simulink model "LKS_1"  (R2018a)
settings: Solver=FixedStepAuto  StartTime=0.0  StopTime=10.0  RelTol=1e-3
values from neighbouring files (symbols this model uses):
  a11 = -2*(cf+cr)/m/v    (= -8.91428571429)    [LKS.m]
  a12 = -1-2*(lf*cf-lr*cr)/m/v/v    (= -0.975808)    [LKS.m]
  a21 = -2*(lf*cf-lr*cr)/iz    (= 12.3270440252)    [LKS.m]
  a22 = -2*(lf*lf*cf+lr*lr*cr)/iz/v    (= -9.16473962264)    [LKS.m]
  b11 = 2*cf/m/v    (= 3.42857142857)    [LKS.m]
  b12 = 0    [LKS.m]
  b21 = 2*lf*cf/iz    (= 94.3396226415)    [LKS.m]
  b22 = 1/iz    (= 0.0062893081761)    [LKS.m]
  dv = 0.814    [LKS.m]
  g1 = 2*(cf+cr)/m/v+2*(lf*lf*cf+lr*lr*cr)/iz/v    (= 18.0790253369)    [LKS.m]
  go = 4*l*l*cf*cr/m/iz/v/v-2*(lf*cf-lr*cr)/iz    (= 93.7259356694)    [LKS.m]
  hm1 = 1/iz    (= 0.0062893081761)    [LKS.m]
  hmo = 2*(cf+cr)/m/iz/v    (= 0.056064690027)    [LKS.m]
  L = 6.31    [LKS.m]
  mydt = 0.01    [LKS.m]
  rw = 0.225    [LKS.m]
  v = vkm/3.6    (= 13.8888888889)    [LKS.m]
libraries: simulink x2
settings Model: Creator=aoki-soya  LastModifiedBy=aoki-soya

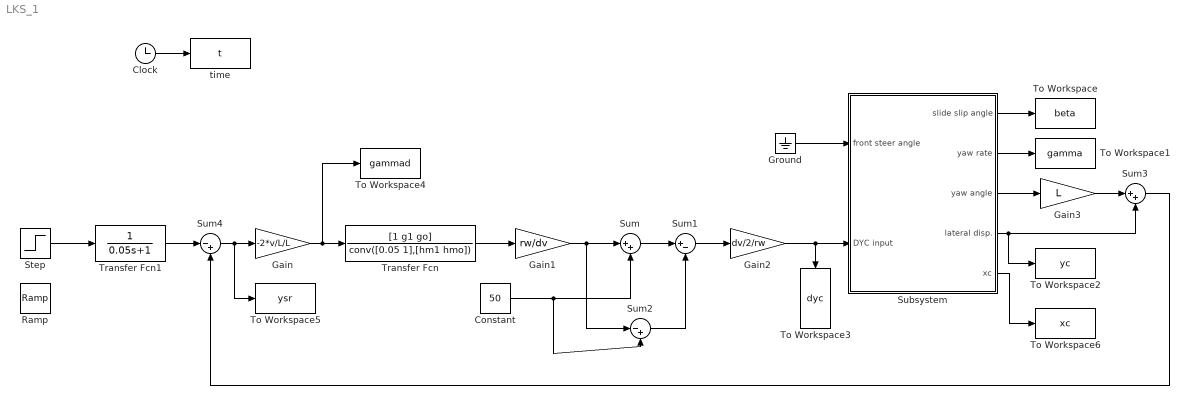
== system LKS_1 ==
  Clock : Clock
      settings: Decimation=1/mydt
  Constant : Constant  Value=50
  Gain : Gain  Gain=-2*v/L/L
  Gain1 : Gain  Gain=rw/dv
  Gain2 : Gain  Gain=dv/2/rw
  Gain3 : Gain  Gain=L
  Ground : Ground
  Ramp : simulink/Sources/Ramp  slope=1  start=1  InitialOutput=0
  Step : Step  SampleTime=mydt
  Subsystem : Subsystem
  Sum : Sum  Inputs=|++
  Sum1 : Sum  Inputs=|+-
  Sum2 : Sum  Inputs=|-+
  Sum3 : Sum  Inputs=|++
  Sum4 : Sum  Inputs=|-+
  To Workspace : ToWorkspace  VariableName=beta  SaveFormat=Timeseries  SampleTime=-1
  To Workspace1 : ToWorkspace  VariableName=gamma  SaveFormat=Timeseries  SampleTime=-1
  To Workspace2 : ToWorkspace  VariableName=yc  SaveFormat=Timeseries  SampleTime=-1
  To Workspace3 : ToWorkspace  VariableName=dyc  SaveFormat=Timeseries  SampleTime=-1
  To Workspace4 : ToWorkspace  VariableName=gammad  SaveFormat=Timeseries  SampleTime=-1
  To Workspace5 : ToWorkspace  VariableName=ysr  SaveFormat=Timeseries  SampleTime=-1
  To Workspace6 : ToWorkspace  VariableName=xc  SaveFormat=Timeseries  SampleTime=-1
  Transfer Fcn : TransferFcn  Numerator=[1 g1 go]  Denominator=conv([0.05 1],[hm1 hmo])
  Transfer Fcn1 : TransferFcn  Denominator=[0.05 1]
  time : ToWorkspace  VariableName=t  SaveFormat=Timeseries  SampleTime=-1
  wires:
  Gain/1 -> To Workspace4/1, Transfer Fcn/1
  Transfer Fcn/1 -> Gain1/1
  Gain1/1 -> Sum2/1, Sum/1
  Sum/1 -> Sum1/1
  Sum2/1 -> Sum1/2
  Constant/1 -> Sum2/2, Sum/2
  Sum1/1 -> Gain2/1
  Gain2/1 -> To Workspace3/1, Subsystem/2(DYC input)
  Ground/1 -> Subsystem/1(front steer angle)
  Clock/1 -> time/1
  Subsystem/3(yaw angle) -> Gain3/1
  Gain3/1 -> Sum3/1
  Sum4/1 -> To Workspace5/1, Gain/1
  Sum3/1 -> Sum4/2
  Subsystem/1(slide slip angle) -> To Workspace/1
  Subsystem/2(yaw rate) -> To Workspace1/1
  Subsystem/4("lateral disp. ") -> To Workspace2/1, Sum3/2
  Subsystem/5("xc ") -> To Workspace6/1
  Transfer Fcn1/1 -> Sum4/1
  Step/1 -> Transfer Fcn1/1

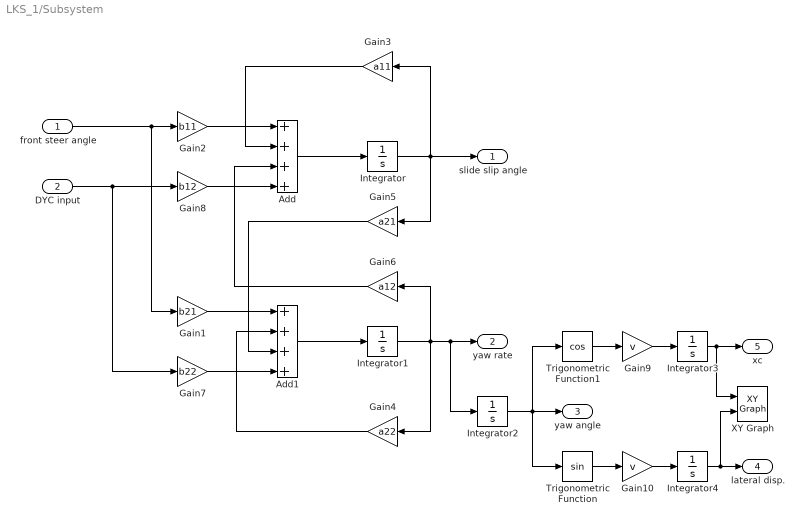
== system LKS_1/Subsystem ==
  front steer angle : Inport
  DYC input : Inport  Port=2
  Add : Sum  Inputs=++++
  Add1 : Sum  Inputs=++++
  Gain1 : Gain  Gain=b21
  Gain10 : Gain  Gain=v
  Gain2 : Gain  Gain=b11
  Gain3 : Gain  Gain=a11
  Gain4 : Gain  Gain=a22
  Gain5 : Gain  Gain=a21
  Gain6 : Gain  Gain=a12
  Gain7 : Gain  Gain=b22
  Gain8 : Gain  Gain=b12
  Gain9 : Gain  Gain=v
  Integrator{,1..4} (5 alike) : Integrator
  Trigonometric Function : Trigonometry
  Trigonometric Function1 : Trigonometry  Operator=cos
  XY Graph : simulink/Sinks/XY Graph  xmin=0  xmax=100  ymin=0  ymax=5  st=-1
  slide slip angle : Outport
  yaw rate : Outport  Port=2
  yaw angle : Outport  Port=3
  "lateral disp. " : Outport  Port=4
  "xc " : Outport  Port=5
  wires:
  Add1/1 -> Integrator1/1
  Integrator1/1 -> Integrator2/1, yaw rate/1, Gain6/1, Gain4/1
  Gain1/1 -> Add1/1
  Gain5/1 -> Add1/3
  Integrator/1 -> slide slip angle/1, Gain5/1, Gain3/1
  front steer angle/1 -> Gain1/1, Gain2/1
  Gain2/1 -> Add/1
  Gain4/1 -> Add1/2
  Add/1 -> Integrator/1
  Gain6/1 -> Add/3
  Gain3/1 -> Add/2
  DYC input/1 -> Gain7/1, Gain8/1
  Gain8/1 -> Add/4
  Gain7/1 -> Add1/4
  Integrator2/1 -> Trigonometric Function1/1, yaw angle/1, Trigonometric Function/1
  Trigonometric Function1/1 -> Gain9/1
  Trigonometric Function/1 -> Gain10/1
  Gain9/1 -> Integrator3/1
  Gain10/1 -> Integrator4/1
  Integrator4/1 -> XY Graph/2, "lateral disp. "/1
  Integrator3/1 -> XY Graph/1, "xc "/1
